simulink model "control_system"  (R2020b)
settings: Solver=FixedStepAuto  StartTime=0.0  StopTime=t_sim  FixedStep=Ts  RelTol=1e-2
values from neighbouring files (symbols this model uses):
  Hp = 10    [main_script.m]
  InitPosX = -2.4980e+03    (= -2498)    [main_script.m]
  InitPosY = -650.5503    [main_script.m]
  InitVelX = V0*cosd(InitYaw)    [main_script.m]
  InitVelY = V0*sind(InitYaw)    [main_script.m]
  InitYaw = 21    [main_script.m]
  lr = 1.592    [main_script.m]
  m = 1625    [main_script.m]
  Ts = 0.1    [main_script.m]
  V0 = 25    [main_script.m]
libraries: neural x856, simulink x1, autolibshared x1, drivingscenarioandsensors x1
(part 31 of 40)

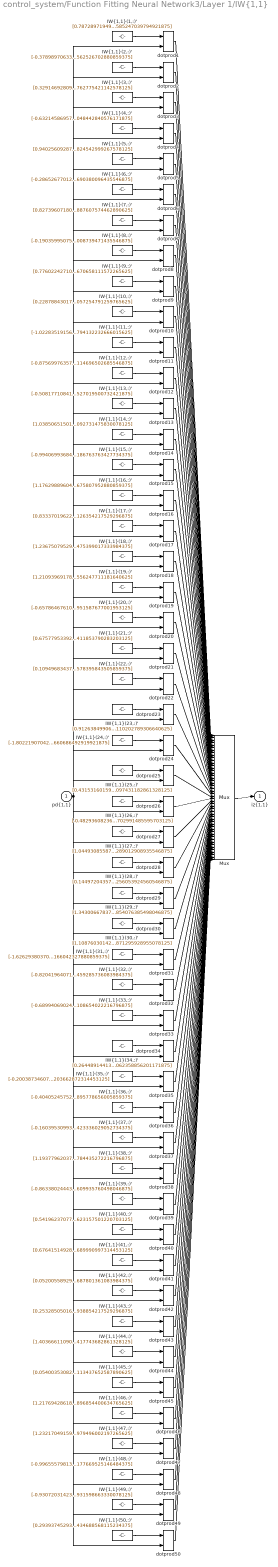
== system control_system/Function Fitting Neural Network3/Layer 1/IW{1,1} ==
  "pd{1,1}" : Inport  PortDimensions=9  SampleTime=0.1
      mask Display: e = 0.06;c1 = [120 230 180]/255;c2 = ([120 230 180]+0)/(256+128);c3 = ([120 230 180]+128)/(256+128);patch([0 1 1 0],[0 0 1 1],c1);patch([0 1 1 1-e 1-e 0+e],[0 0 1 1-e 0+e 0+e],c2);patch([0 0 1 1-e 0+e 0+e],[0 1 1 1-e 1-e 0+e],c3);plot([0 1 1 0 0],[0 0 1 1 0]);
  "IW{1,1}(1,:)'" : Constant  Value=[0.78728971949492476678500452180742286145687103271484375;0.352797731152850790881103648644057102501392364501953125;0.8265331890279414839284299887367524206638336181640625;-0.1863624056692552988234723443383700214326381683349609375;-0.7777782099348835576080318787717260420322418212890625;-0.5426301554164287832549007362104021012783050537109375;-0.6404421601342054071182019470143131911754608154296875;-0.99503704364510625612894045843859203159809112548828125;-0.948568198681023044827043122495524585247039794921875]
      mask Display: e = 0.06;c1 = [120 150 230]/255;c2 = ([120 150 230]+0)/383;c3 = ([120 150 230]+128)/383;patch([0 1 1 0],[0 0 1 1],c1);patch([0 1 1 1-e 1-e 0+e],[0 0 1 1-e 0+e 0+e],c2);patch([0 0 1 1-e 0+e 0+e],[0 1 1 1-e 1-e 0+e],c3);plot([0 1 1 0 0],[0 0 1 1 0]);disp('Weights');
  "IW{1,1}(10,:)'" : Constant  Value=[0.2287884301751469673380512404037290252745151519775390625;-0.0631161080977170330097436590222059749066829681396484375;1.0790651138932052521823834467795677483081817626953125;-0.738474613619092057348325397470034658908843994140625;0.0118735259410528148915631163617945276200771331787109375;1.1493716684892592017064316678442992269992828369140625;0.8580199635066418917261898968718014657497406005859375;0.1895198552495412636087479540947242639958858489990234375;-0.9068559161380724820133991670445539057254791259765625]
      mask Display: e = 0.06;c1 = [120 150 230]/255;c2 = ([120 150 230]+0)/383;c3 = ([120 150 230]+128)/383;patch([0 1 1 0],[0 0 1 1],c1);patch([0 1 1 1-e 1-e 0+e],[0 0 1 1-e 0+e 0+e],c2);patch([0 0 1 1-e 0+e 0+e],[0 1 1 1-e 1-e 0+e],c3);plot([0 1 1 0 0],[0 0 1 1 0]);disp('Weights');
  "IW{1,1}(11,:)'" : Constant  Value=[-1.0228351915632918345266944015747867524623870849609375;-0.021838659789676147238157710717132431454956531524658203125;-0.415484340574546917590481598381302319467067718505859375;-1.060341109567944695157848400413058698177337646484375;1.2054314419390748103211308261961676180362701416015625;-1.0443864348574185552109838681644760072231292724609375;-0.8779072415157027631238406684133224189281463623046875;0.349684007816375153065990843970212154090404510498046875;0.0266467695099608693765080857929206104017794132232666015625]
      mask Display: e = 0.06;c1 = [120 150 230]/255;c2 = ([120 150 230]+0)/383;c3 = ([120 150 230]+128)/383;patch([0 1 1 0],[0 0 1 1],c1);patch([0 1 1 1-e 1-e 0+e],[0 0 1 1-e 0+e 0+e],c2);patch([0 0 1 1-e 0+e 0+e],[0 1 1 1-e 1-e 0+e],c3);plot([0 1 1 0 0],[0 0 1 1 0]);disp('Weights');
  "IW{1,1}(12,:)'" : Constant  Value=[-0.875699763578115408790836227126419544219970703125;-0.242759821567909594985934518263093195855617523193359375;1.2159085613981057694132914548390544950962066650390625;0.4044163132053437692547959159128367900848388671875;1.07575999978741077001131998258642852306365966796875;1.8004386650346335674299780293949879705905914306640625;-0.9917103190571128212837948012747801840305328369140625;1.3494754673529085753358458532602526247501373291015625;-0.9851225876669171821475856631877832114696502685546875]
      mask Display: e = 0.06;c1 = [120 150 230]/255;c2 = ([120 150 230]+0)/383;c3 = ([120 150 230]+128)/383;patch([0 1 1 0],[0 0 1 1],c1);patch([0 1 1 1-e 1-e 0+e],[0 0 1 1-e 0+e 0+e],c2);patch([0 0 1 1-e 0+e 0+e],[0 1 1 1-e 1-e 0+e],c3);plot([0 1 1 0 0],[0 0 1 1 0]);disp('Weights');
  "IW{1,1}(13,:)'" : Constant  Value=[-0.50817710841719809788941120132221840322017669677734375;1.08852825196150693187746583134867250919342041015625;-1.3310195810328024901281196434865705668926239013671875;-1.041602136557479685308180705760605633258819580078125;-0.97705606452752336021916335084824822843074798583984375;-0.6948444334830787827428366654203273355960845947265625;-0.362171807844527238184895168160437606275081634521484375;0.1192369383747513833515796477513504214584827423095703125;0.290041715158442847677378040316398255527019500732421875]
      mask Display: e = 0.06;c1 = [120 150 230]/255;c2 = ([120 150 230]+0)/383;c3 = ([120 150 230]+128)/383;patch([0 1 1 0],[0 0 1 1],c1);patch([0 1 1 1-e 1-e 0+e],[0 0 1 1-e 0+e 0+e],c2);patch([0 0 1 1-e 0+e 0+e],[0 1 1 1-e 1-e 0+e],c3);plot([0 1 1 0 0],[0 0 1 1 0]);disp('Weights');
  "IW{1,1}(14,:)'" : Constant  Value=[1.0385065150165868619325237887096591293811798095703125;-0.0299341860920388953826165590044183772988617420196533203125;0.7451840663694848654330371573450975120067596435546875;-0.53186345138759227868519019466475583612918853759765625;-0.032742045322379752236852112901033251546323299407958984375;1.2450800939264377031889807767583988606929779052734375;1.1805822712498803550573711618199013173580169677734375;0.3130863479653560599302863920456729829311370849609375;0.2068094194929717410946778954894398339092731475830078125]
      mask Display: e = 0.06;c1 = [120 150 230]/255;c2 = ([120 150 230]+0)/383;c3 = ([120 150 230]+128)/383;patch([0 1 1 0],[0 0 1 1],c1);patch([0 1 1 1-e 1-e 0+e],[0 0 1 1-e 0+e 0+e],c2);patch([0 0 1 1-e 0+e 0+e],[0 1 1 1-e 1-e 0+e],c3);plot([0 1 1 0 0],[0 0 1 1 0]);disp('Weights');
  "IW{1,1}(15,:)'" : Constant  Value=[-0.99406993684322342286208140649250708520412445068359375;-0.334299503704392264591405137252877466380596160888671875;0.8578503214193753390048868823214434087276458740234375;-0.297048476488083579294396940895239822566509246826171875;-1.0704668818161728882643046745215542614459991455078125;-0.60807184451268858627059898935840465128421783447265625;-0.66391007727095929791261141872382722795009613037109375;1.66801104611655848231066556763835251331329345703125;-0.38683369041100712504288594573154114186763763427734375]
      mask Display: e = 0.06;c1 = [120 150 230]/255;c2 = ([120 150 230]+0)/383;c3 = ([120 150 230]+128)/383;patch([0 1 1 0],[0 0 1 1],c1);patch([0 1 1 1-e 1-e 0+e],[0 0 1 1-e 0+e 0+e],c2);patch([0 0 1 1-e 0+e 0+e],[0 1 1 1-e 1-e 0+e],c3);plot([0 1 1 0 0],[0 0 1 1 0]);disp('Weights');
  "IW{1,1}(16,:)'" : Constant  Value=[1.176298896048470599140500780777074396610260009765625;-0.8988232289150623888218660795246250927448272705078125;0.09615576773442553737414328907107119448482990264892578125;0.48788471027654944922602453516446985304355621337890625;1.037047709591436994713831154513172805309295654296875;0.55055285364358841349030626588501036167144775390625;-0.17909145298814654889696384998387657105922698974609375;0.81145522342693199302487983004539273679256439208984375;0.021295651159626081960762888911631307564675807952880859375]
      mask Display: e = 0.06;c1 = [120 150 230]/255;c2 = ([120 150 230]+0)/383;c3 = ([120 150 230]+128)/383;patch([0 1 1 0],[0 0 1 1],c1);patch([0 1 1 1-e 1-e 0+e],[0 0 1 1-e 0+e 0+e],c2);patch([0 0 1 1-e 0+e 0+e],[0 1 1 1-e 1-e 0+e],c3);plot([0 1 1 0 0],[0 0 1 1 0]);disp('Weights');
  "IW{1,1}(17,:)'" : Constant  Value=[0.83337019622696739684641897838446311652660369873046875;-0.36366566717185555557279030836070887744426727294921875;-0.96023270638495639150988836263422854244709014892578125;1.2783373677316156591388107699458487331867218017578125;0.8916276331235633012539665287476964294910430908203125;-0.6694170731239468263851222218363545835018157958984375;-0.925192516466152081733298473409377038478851318359375;-1.052006199283979537284494654159061610698699951171875;-0.7764706210752112536255253871786408126354217529296875]
      mask Display: e = 0.06;c1 = [120 150 230]/255;c2 = ([120 150 230]+0)/383;c3 = ([120 150 230]+128)/383;patch([0 1 1 0],[0 0 1 1],c1);patch([0 1 1 1-e 1-e 0+e],[0 0 1 1-e 0+e 0+e],c2);patch([0 0 1 1-e 0+e 0+e],[0 1 1 1-e 1-e 0+e],c3);plot([0 1 1 0 0],[0 0 1 1 0]);disp('Weights');
  "IW{1,1}(18,:)'" : Constant  Value=[1.236750795296624350072534070932306349277496337890625;-0.55986879173246772989358532868209294974803924560546875;-1.3800915711518084716402654521516524255275726318359375;1.3289904008938917545634694761247374117374420166015625;0.60327067881495100021282951274770312011241912841796875;-0.4150673095081656160942884525866247713565826416015625;-0.019363883654753132057546594069208367727696895599365234375;0.1294585767502997308842083157287561334669589996337890625;-0.74106167458830130012614745282917283475399017333984375]
      mask Display: e = 0.06;c1 = [120 150 230]/255;c2 = ([120 150 230]+0)/383;c3 = ([120 150 230]+128)/383;patch([0 1 1 0],[0 0 1 1],c1);patch([0 1 1 1-e 1-e 0+e],[0 0 1 1-e 0+e 0+e],c2);patch([0 0 1 1-e 0+e 0+e],[0 1 1 1-e 1-e 0+e],c3);plot([0 1 1 0 0],[0 0 1 1 0]);disp('Weights');
  "IW{1,1}(19,:)'" : Constant  Value=[1.2109396917827270900858138702460564672946929931640625;0.1326857718800483476595530873964889906346797943115234375;-0.465325794397773273569640650748624466359615325927734375;-0.53881885042031452126565227445098571479320526123046875;-0.8667873778604668899561147554777562618255615234375;-0.1324460904740631661535843477395246736705303192138671875;-0.6026871578635122350675601410330273211002349853515625;0.2041421396899969764593407717256923206150531768798828125;1.1937448304855708958172044731327332556247711181640625]
      mask Display: e = 0.06;c1 = [120 150 230]/255;c2 = ([120 150 230]+0)/383;c3 = ([120 150 230]+128)/383;patch([0 1 1 0],[0 0 1 1],c1);patch([0 1 1 1-e 1-e 0+e],[0 0 1 1-e 0+e 0+e],c2);patch([0 0 1 1-e 0+e 0+e],[0 1 1 1-e 1-e 0+e],c3);plot([0 1 1 0 0],[0 0 1 1 0]);disp('Weights');
  "IW{1,1}(2,:)'" : Constant  Value=[-0.378989706335502607448262324396637268364429473876953125;-1.1437056077678295906707717222161591053009033203125;0.330358132573418228350448089258861728012561798095703125;-0.476080786756290341710240454631275497376918792724609375;-0.4363164287721887912852025692700408399105072021484375;-0.63772136886470409677940551773644983768463134765625;-1.174846406412093369198146319831721484661102294921875;-0.77474853404004928592030410072766244411468505859375;-0.2296675389268350853111400056150159798562526702880859375]
      mask Display: e = 0.06;c1 = [120 150 230]/255;c2 = ([120 150 230]+0)/383;c3 = ([120 150 230]+128)/383;patch([0 1 1 0],[0 0 1 1],c1);patch([0 1 1 1-e 1-e 0+e],[0 0 1 1-e 0+e 0+e],c2);patch([0 0 1 1-e 0+e 0+e],[0 1 1 1-e 1-e 0+e],c3);plot([0 1 1 0 0],[0 0 1 1 0]);disp('Weights');
  "IW{1,1}(20,:)'" : Constant  Value=[-0.65786467610956089746565567111247219145298004150390625;1.362933438760308479942295889486558735370635986328125;0.210346089395960611501124049027566798031330108642578125;-0.7030459458053137655753062063013203442096710205078125;0.63733479975609863554808498520287685096263885498046875;-0.7983018398063055354185735268401913344860076904296875;0.648857536128780498785317831789143383502960205078125;0.8394757099670868694119008068810217082500457763671875;-0.52279242792795888039592000495758838951587677001953125]
      mask Display: e = 0.06;c1 = [120 150 230]/255;c2 = ([120 150 230]+0)/383;c3 = ([120 150 230]+128)/383;patch([0 1 1 0],[0 0 1 1],c1);patch([0 1 1 1-e 1-e 0+e],[0 0 1 1-e 0+e 0+e],c2);patch([0 0 1 1-e 0+e 0+e],[0 1 1 1-e 1-e 0+e],c3);plot([0 1 1 0 0],[0 0 1 1 0]);disp('Weights');
  "IW{1,1}(21,:)'" : Constant  Value=[0.67577953392096989926329797526705078780651092529296875;0.8608869950072242094307739534997381269931793212890625;-0.11469898640935526079598361093303537927567958831787109375;1.1193380407867741244132275824085809290409088134765625;-0.9683403733384603473410834340029396116733551025390625;0.027391112412877567650060228743313928134739398956298828125;-1.209926726376689298803057681652717292308807373046875;-0.268730649947182820280744408591999672353267669677734375;-0.8212758063260576779640587119502015411853790283203125]
      mask Display: e = 0.06;c1 = [120 150 230]/255;c2 = ([120 150 230]+0)/383;c3 = ([120 150 230]+128)/383;patch([0 1 1 0],[0 0 1 1],c1);patch([0 1 1 1-e 1-e 0+e],[0 0 1 1-e 0+e 0+e],c2);patch([0 0 1 1-e 0+e 0+e],[0 1 1 1-e 1-e 0+e],c3);plot([0 1 1 0 0],[0 0 1 1 0]);disp('Weights');
  "IW{1,1}(22,:)'" : Constant  Value=[0.10949683437770142691025654357872554101049900054931640625;0.87280978510004214587780779766035266220569610595703125;-1.0316109104847950295180680768680758774280548095703125;0.9729898005523214266077047795988619327545166015625;1.0304574213938497706521957297809422016143798828125;-0.341709897445362897894227671713451854884624481201171875;-0.6454097992064846689430623882799409329891204833984375;-0.656223486076811468592495657503604888916015625;0.2604852028852560064109411541721783578395843505859375]
      mask Display: e = 0.06;c1 = [120 150 230]/255;c2 = ([120 150 230]+0)/383;c3 = ([120 150 230]+128)/383;patch([0 1 1 0],[0 0 1 1],c1);patch([0 1 1 1-e 1-e 0+e],[0 0 1 1-e 0+e 0+e],c2);patch([0 0 1 1-e 0+e 0+e],[0 1 1 1-e 1-e 0+e],c3);plot([0 1 1 0 0],[0 0 1 1 0]);disp('Weights');
  "IW{1,1}(23,:)'" : Constant  Value=[0.912638499065945740795768870157189667224884033203125;0.62788843775751457254585830014548264443874359130859375;-0.11544045247414332078239596057755989022552967071533203125;0.72876930448921173333332035326748155057430267333984375;0.0930837705597644948785074348052148707211017608642578125;0.70534305814777942256199594339705072343349456787109375;0.79724782708528263430736160444212146103382110595703125;1.5542498026142135270077915265574119985103607177734375;-0.0814864679916317558028282519444474019110202789306640625]
      mask Display: e = 0.06;c1 = [120 150 230]/255;c2 = ([120 150 230]+0)/383;c3 = ([120 150 230]+128)/383;patch([0 1 1 0],[0 0 1 1],c1);patch([0 1 1 1-e 1-e 0+e],[0 0 1 1-e 0+e 0+e],c2);patch([0 0 1 1-e 0+e 0+e],[0 1 1 1-e 1-e 0+e],c3);plot([0 1 1 0 0],[0 0 1 1 0]);disp('Weights');
  "IW{1,1}(24,:)'" : Constant  Value=[-1.802219070424301516908371922909282147884368896484375;-0.340985615024179289367367573504452593624591827392578125;-0.5377858984214862747563756784074939787387847900390625;-1.515689046597109790326385336811654269695281982421875;0.51434483958638843592581224584137089550495147705078125;-0.1567876230668934223189125987119041383266448974609375;0.351340893838307299912315784240490756928920745849609375;1.368712963354658196379887158400379121303558349609375;-0.66279873807852573985854860438848845660686492919921875]
      mask Display: e = 0.06;c1 = [120 150 230]/255;c2 = ([120 150 230]+0)/383;c3 = ([120 150 230]+128)/383;patch([0 1 1 0],[0 0 1 1],c1);patch([0 1 1 1-e 1-e 0+e],[0 0 1 1-e 0+e 0+e],c2);patch([0 0 1 1-e 0+e 0+e],[0 1 1 1-e 1-e 0+e],c3);plot([0 1 1 0 0],[0 0 1 1 0]);disp('Weights');
  "IW{1,1}(25,:)'" : Constant  Value=[0.43153160159828851671903748865588568150997161865234375;-0.77360038084864990448608068618341349065303802490234375;-1.18295318629940737764627556316554546356201171875;-0.433606385185640819113217503399937413632869720458984375;-0.2244183057689046467686466712621040642261505126953125;-0.7321900135293717415407854787190444767475128173828125;-0.451425117568696077086087825591675937175750732421875;1.1856571858869806579406258606468327343463897705078125;0.04425940707458864142864740642835386097431182861328125]
      mask Display: e = 0.06;c1 = [120 150 230]/255;c2 = ([120 150 230]+0)/383;c3 = ([120 150 230]+128)/383;patch([0 1 1 0],[0 0 1 1],c1);patch([0 1 1 1-e 1-e 0+e],[0 0 1 1-e 0+e 0+e],c2);patch([0 0 1 1-e 0+e 0+e],[0 1 1 1-e 1-e 0+e],c3);plot([0 1 1 0 0],[0 0 1 1 0]);disp('Weights');
  "IW{1,1}(26,:)'" : Constant  Value=[-0.482936082364363639118920445980620570480823516845703125;-0.9309568746589584886663715224131010472774505615234375;-0.1503448104672455432062605495957541279494762420654296875;-1.198029994378850826564075759961269795894622802734375;0.259575336572962889203353142875130288302898406982421875;0.27904855673582318331682472489774227142333984375;-0.50645491575020995522748989969841204583644866943359375;0.62272600542499245701577592626563273370265960693359375;-1.202204106531607141761242019128985702991485595703125]
      mask Display: e = 0.06;c1 = [120 150 230]/255;c2 = ([120 150 230]+0)/383;c3 = ([120 150 230]+128)/383;patch([0 1 1 0],[0 0 1 1],c1);patch([0 1 1 1-e 1-e 0+e],[0 0 1 1-e 0+e 0+e],c2);patch([0 0 1 1-e 0+e 0+e],[0 1 1 1-e 1-e 0+e],c3);plot([0 1 1 0 0],[0 0 1 1 0]);disp('Weights');
  "IW{1,1}(27,:)'" : Constant  Value=[1.044930855879160791488402537652291357517242431640625;-0.860944056842925409256395141710527241230010986328125;0.887825241736790449209593134582974016666412353515625;0.427993292709983375043947262383881025016307830810546875;-0.457723346034051792319274909459636546671390533447265625;-0.55042069308471652799852336102048866450786590576171875;-0.87332778872113137058619258823455311357975006103515625;-0.6366049352812364059417404860141687095165252685546875;0.70842194831802440813106613859417848289012908935546875]
      mask Display: e = 0.06;c1 = [120 150 230]/255;c2 = ([120 150 230]+0)/383;c3 = ([120 150 230]+128)/383;patch([0 1 1 0],[0 0 1 1],c1);patch([0 1 1 1-e 1-e 0+e],[0 0 1 1-e 0+e 0+e],c2);patch([0 0 1 1-e 0+e 0+e],[0 1 1 1-e 1-e 0+e],c3);plot([0 1 1 0 0],[0 0 1 1 0]);disp('Weights');
  "IW{1,1}(28,:)'" : Constant  Value=[0.144972043576537090725508960531442426145076751708984375;0.1541953436889172690538174492758116684854030609130859375;-0.77822769384765655420466146097169257700443267822265625;-1.0198035630015633845601996654295362532138824462890625;-0.51659780456091886069458496422157622873783111572265625;1.39939210966581573103439950500614941120147705078125;0.295882266856562381462936173193156719207763671875;1.0654792493903155747858590984833426773548126220703125;0.641300014924847783248651467147283256053924560546875]
      mask Display: e = 0.06;c1 = [120 150 230]/255;c2 = ([120 150 230]+0)/383;c3 = ([120 150 230]+128)/383;patch([0 1 1 0],[0 0 1 1],c1);patch([0 1 1 1-e 1-e 0+e],[0 0 1 1-e 0+e 0+e],c2);patch([0 0 1 1-e 0+e 0+e],[0 1 1 1-e 1-e 0+e],c3);plot([0 1 1 0 0],[0 0 1 1 0]);disp('Weights');
  "IW{1,1}(29,:)'" : Constant  Value=[1.3430066783716971823281483011669479310512542724609375;-0.8969042973177840938348026611492969095706939697265625;-1.076092110823586356360692661837674677371978759765625;0.244234872350051868128417709158384241163730621337890625;0.495632237070989634108997279327013529837131500244140625;-0.31289164058760310371809509888407774269580841064453125;-0.912975658702446679626518744044005870819091796875;0.0809968678519148443939457138185389339923858642578125;0.397991863783186516911882790736854076385498046875]
      mask Display: e = 0.06;c1 = [120 150 230]/255;c2 = ([120 150 230]+0)/383;c3 = ([120 150 230]+128)/383;patch([0 1 1 0],[0 0 1 1],c1);patch([0 1 1 1-e 1-e 0+e],[0 0 1 1-e 0+e 0+e],c2);patch([0 0 1 1-e 0+e 0+e],[0 1 1 1-e 1-e 0+e],c3);plot([0 1 1 0 0],[0 0 1 1 0]);disp('Weights');
  "IW{1,1}(3,:)'" : Constant  Value=[0.3291469280906638150696608136058785021305084228515625;0.62737660797549354985136460527428425848484039306640625;0.78915346814299869304676349202054552733898162841796875;-0.90552136457697385285570135238231159746646881103515625;0.257465585146909037295159805580624379217624664306640625;0.221382776389055069277134180083521641790866851806640625;1.4252850062237729655834073128062300384044647216796875;-0.69989724392903751581940241521806456148624420166015625;0.20729749308358613735236986030940897762775421142578125]
      mask Display: e = 0.06;c1 = [120 150 230]/255;c2 = ([120 150 230]+0)/383;c3 = ([120 150 230]+128)/383;patch([0 1 1 0],[0 0 1 1],c1);patch([0 1 1 1-e 1-e 0+e],[0 0 1 1-e 0+e 0+e],c2);patch([0 0 1 1-e 0+e 0+e],[0 1 1 1-e 1-e 0+e],c3);plot([0 1 1 0 0],[0 0 1 1 0]);disp('Weights');
  "IW{1,1}(30,:)'" : Constant  Value=[1.108760301421545246824962305254302918910980224609375;0.86207759324852251126003466197289526462554931640625;-0.11670050893409382453125289202944259159266948699951171875;1.2386076034523905153861278449767269194126129150390625;-1.0526726240503554432592636658228002488613128662109375;1.1240606375888670953600012580864131450653076171875;0.92538279206566487200547044267295859754085540771484375;-1.3685636484095333731403343335841782391071319580078125;-0.69779752491048718798793970563565380871295928955078125]
      mask Display: e = 0.06;c1 = [120 150 230]/255;c2 = ([120 150 230]+0)/383;c3 = ([120 150 230]+128)/383;patch([0 1 1 0],[0 0 1 1],c1);patch([0 1 1 1-e 1-e 0+e],[0 0 1 1-e 0+e 0+e],c2);patch([0 0 1 1-e 0+e 0+e],[0 1 1 1-e 1-e 0+e],c3);plot([0 1 1 0 0],[0 0 1 1 0]);disp('Weights');
  "IW{1,1}(31,:)'" : Constant  Value=[-1.6262938037064917917717821183032356202602386474609375;-0.347778459901182335212155294357216916978359222412109375;0.83231871936962031899298608550452627241611480712890625;-1.122571461750564214554515274357981979846954345703125;1.039097624203837444412101831403560936450958251953125;-0.81297977449732883314936771057546138763427734375;1.113158335871994975008192341192625463008880615234375;-0.1408702915339343775258384994231164455413818359375;-0.031547675269102126716092016067705117166042327880859375]
      mask Display: e = 0.06;c1 = [120 150 230]/255;c2 = ([120 150 230]+0)/383;c3 = ([120 150 230]+128)/383;patch([0 1 1 0],[0 0 1 1],c1);patch([0 1 1 1-e 1-e 0+e],[0 0 1 1-e 0+e 0+e],c2);patch([0 0 1 1-e 0+e 0+e],[0 1 1 1-e 1-e 0+e],c3);plot([0 1 1 0 0],[0 0 1 1 0]);disp('Weights');
  "IW{1,1}(32,:)'" : Constant  Value=[-0.82041964071189787954807570713455788791179656982421875;-0.32324692831648238477981749383616261184215545654296875;0.6458209200762670132434095648932270705699920654296875;0.23384694042951437165100969650666229426860809326171875;-1.291500322629459684975472555379383265972137451171875;-1.5974304191525749985203219694085419178009033203125;0.444373258878406340866007440126850269734859466552734375;1.57149179936640681631843108334578573703765869140625;0.269491929332904278648896934100775979459285736083984375]
      mask Display: e = 0.06;c1 = [120 150 230]/255;c2 = ([120 150 230]+0)/383;c3 = ([120 150 230]+128)/383;patch([0 1 1 0],[0 0 1 1],c1);patch([0 1 1 1-e 1-e 0+e],[0 0 1 1-e 0+e 0+e],c2);patch([0 0 1 1-e 0+e 0+e],[0 1 1 1-e 1-e 0+e],c3);plot([0 1 1 0 0],[0 0 1 1 0]);disp('Weights');
  "IW{1,1}(33,:)'" : Constant  Value=[-0.689940690243980636608966960920952260494232177734375;-1.4101558786294583480724895707680843770503997802734375;0.1630877244993971242337238436448387801647186279296875;-1.7669812635201058714784494441119022667407989501953125;-0.482624421254764346400634167366661131381988525390625;-0.9612055055403947445569201590842567384243011474609375;1.3015624416982609634629852735088206827640533447265625;0.0875738032916208719580453134767594747245311737060546875;0.040220794334714475570802250103952246718108654022216796875]
      mask Display: e = 0.06;c1 = [120 150 230]/255;c2 = ([120 150 230]+0)/383;c3 = ([120 150 230]+128)/383;patch([0 1 1 0],[0 0 1 1],c1);patch([0 1 1 1-e 1-e 0+e],[0 0 1 1-e 0+e 0+e],c2);patch([0 0 1 1-e 0+e 0+e],[0 1 1 1-e 1-e 0+e],c3);plot([0 1 1 0 0],[0 0 1 1 0]);disp('Weights');
  "IW{1,1}(34,:)'" : Constant  Value=[0.264489144130551523392824719849159009754657745361328125;-0.11668913145246741225324882407221593894064426422119140625;0.60220127682401358715225114792701788246631622314453125;1.7380237708569612475884014202165417373180389404296875;0.6104130038792170420691718391026370227336883544921875;-1.70710467850310987358852798934094607830047607421875;-0.92955480038042848089929748311988078057765960693359375;1.5937912860225769140498641718295402824878692626953125;1.4518733032150279438354800731758587062358856201171875]
      mask Display: e = 0.06;c1 = [120 150 230]/255;c2 = ([120 150 230]+0)/383;c3 = ([120 150 230]+128)/383;patch([0 1 1 0],[0 0 1 1],c1);patch([0 1 1 1-e 1-e 0+e],[0 0 1 1-e 0+e 0+e],c2);patch([0 0 1 1-e 0+e 0+e],[0 1 1 1-e 1-e 0+e],c3);plot([0 1 1 0 0],[0 0 1 1 0]);disp('Weights');
  "IW{1,1}(35,:)'" : Constant  Value=[-0.200387346072296856913652618459309451282024383544921875;0.478387526639784843585090357009903527796268463134765625;1.19705813553185880238061145064420998096466064453125;-1.525560920857229607605631827027536928653717041015625;-1.11857885098643095034276484511792659759521484375;2.28596493044082382795068042469210922718048095703125;-0.32697021581169305459724228057893924415111541748046875;0.1161743373023399750199047275600605644285678863525390625;0.9455134287433129003375142929144203662872314453125]
      mask Display: e = 0.06;c1 = [120 150 230]/255;c2 = ([120 150 230]+0)/383;c3 = ([120 150 230]+128)/383;patch([0 1 1 0],[0 0 1 1],c1);patch([0 1 1 1-e 1-e 0+e],[0 0 1 1-e 0+e 0+e],c2);patch([0 0 1 1-e 0+e 0+e],[0 1 1 1-e 1-e 0+e],c3);plot([0 1 1 0 0],[0 0 1 1 0]);disp('Weights');
  "IW{1,1}(36,:)'" : Constant  Value=[-0.4040524575299941911765699842362664639949798583984375;0.56950173003886794820260774940834380686283111572265625;-0.309069682024796510422248729810235090553760528564453125;1.174907768493887783023410520399920642375946044921875;-0.76016435248717650896566055962466634809970855712890625;0.463070298319331830061429400302586145699024200439453125;-0.71977379111322481453072441581753082573413848876953125;0.1662797156150146171693648966538603417575359344482421875;1.231310054411932863871470544836483895778656005859375]
      mask Display: e = 0.06;c1 = [120 150 230]/255;c2 = ([120 150 230]+0)/383;c3 = ([120 150 230]+128)/383;patch([0 1 1 0],[0 0 1 1],c1);patch([0 1 1 1-e 1-e 0+e],[0 0 1 1-e 0+e 0+e],c2);patch([0 0 1 1-e 0+e 0+e],[0 1 1 1-e 1-e 0+e],c3);plot([0 1 1 0 0],[0 0 1 1 0]);disp('Weights');
  "IW{1,1}(37,:)'" : Constant  Value=[-0.160395309938668961802221701873349957168102264404296875;0.410351798316771709806971557554788887500762939453125;1.0788402606665403737906672176904976367950439453125;-0.32839166335755642922578090292518027126789093017578125;-1.0325028530439583906996858786442317068576812744140625;-0.33651519126705686790756999471341259777545928955078125;0.00718425054981363005179861858096046489663422107696533203125;-0.87535165476770548931284565696842037141323089599609375;0.93976986860059719131044175810529850423336029052734375]
      mask Display: e = 0.06;c1 = [120 150 230]/255;c2 = ([120 150 230]+0)/383;c3 = ([120 150 230]+128)/383;patch([0 1 1 0],[0 0 1 1],c1);patch([0 1 1 1-e 1-e 0+e],[0 0 1 1-e 0+e 0+e],c2);patch([0 0 1 1-e 0+e 0+e],[0 1 1 1-e 1-e 0+e],c3);plot([0 1 1 0 0],[0 0 1 1 0]);disp('Weights');
  "IW{1,1}(38,:)'" : Constant  Value=[1.1937796203738368916447143419645726680755615234375;1.230789293167344755630665531498380005359649658203125;0.07832258154244080283756801463823649100959300994873046875;1.5392943653869954889756854754523374140262603759765625;1.5136918318591983112497700858511961996555328369140625;-0.241736218705538796758247599427704699337482452392578125;0.2867327195668918360382804166874848306179046630859375;-1.2139662037220404489090697097708471119403839111328125;0.79571289507152431763614686133223585784435272216796875]
      mask Display: e = 0.06;c1 = [120 150 230]/255;c2 = ([120 150 230]+0)/383;c3 = ([120 150 230]+128)/383;patch([0 1 1 0],[0 0 1 1],c1);patch([0 1 1 1-e 1-e 0+e],[0 0 1 1-e 0+e 0+e],c2);patch([0 0 1 1-e 0+e 0+e],[0 1 1 1-e 1-e 0+e],c3);plot([0 1 1 0 0],[0 0 1 1 0]);disp('Weights');
  "IW{1,1}(39,:)'" : Constant  Value=[-0.86338024443859662238054397676023654639720916748046875;0.86905909058558783453207752245361916720867156982421875;0.578888775818624079505525514832697808742523193359375;-1.474862708423287482872865439276210963726043701171875;1.095471724648996225681685245945118367671966552734375;-0.70623810094509276158447619309299625456333160400390625;-1.1869666187459351203159485521609894931316375732421875;0.206434423646733034019007391179911792278289794921875;-0.91825459226975592041952722865971736609935760498046875]
      mask Display: e = 0.06;c1 = [120 150 230]/255;c2 = ([120 150 230]+0)/383;c3 = ([120 150 230]+128)/383;patch([0 1 1 0],[0 0 1 1],c1);patch([0 1 1 1-e 1-e 0+e],[0 0 1 1-e 0+e 0+e],c2);patch([0 0 1 1-e 0+e 0+e],[0 1 1 1-e 1-e 0+e],c3);plot([0 1 1 0 0],[0 0 1 1 0]);disp('Weights');
  "IW{1,1}(4,:)'" : Constant  Value=[-0.6321458695752950607271714034141041338443756103515625;0.54688250895527812378560383876902051270008087158203125;0.1788397574811165513519739533876418136060237884521484375;0.59342891536845499000918380261282436549663543701171875;0.76115013925244967563088493989198468625545501708984375;1.3158823761126641205265741518815048038959503173828125;1.2724410126391259012734735733829438686370849609375;1.7966390556129059330459085686015896499156951904296875;-0.0220531766669407151837400959948354284279048442840576171875]
      mask Display: e = 0.06;c1 = [120 150 230]/255;c2 = ([120 150 230]+0)/383;c3 = ([120 150 230]+128)/383;patch([0 1 1 0],[0 0 1 1],c1);patch([0 1 1 1-e 1-e 0+e],[0 0 1 1-e 0+e 0+e],c2);patch([0 0 1 1-e 0+e 0+e],[0 1 1 1-e 1-e 0+e],c3);plot([0 1 1 0 0],[0 0 1 1 0]);disp('Weights');
  "IW{1,1}(40,:)'" : Constant  Value=[0.5419623707778138399504541666829027235507965087890625;0.1950556215816010297015026253575342707335948944091796875;1.078199970146870523279858389287255704402923583984375;-1.674137574591714194838232288020662963390350341796875;-0.7880522431413308215297774950158782303333282470703125;0.68010644380544338361005429760552942752838134765625;0.4078215424324758142660130033618770539760589599609375;-2.306607321515167452474770470871590077877044677734375;-0.12174585245644194142489169507825863547623157501220703125]
      mask Display: e = 0.06;c1 = [120 150 230]/255;c2 = ([120 150 230]+0)/383;c3 = ([120 150 230]+128)/383;patch([0 1 1 0],[0 0 1 1],c1);patch([0 1 1 1-e 1-e 0+e],[0 0 1 1-e 0+e 0+e],c2);patch([0 0 1 1-e 0+e 0+e],[0 1 1 1-e 1-e 0+e],c3);plot([0 1 1 0 0],[0 0 1 1 0]);disp('Weights');
  "IW{1,1}(41,:)'" : Constant  Value=[0.67641514928419399499404107700684107840061187744140625;-0.8238474701929126009503079330897890031337738037109375;0.7852656164367346480759124460746534168720245361328125;-1.104985223708661923325280440622009336948394775390625;0.8669948164997738349057954110321588814258575439453125;-0.1704696961773134178397270943605690263211727142333984375;0.568046795494847600593857350759208202362060546875;-0.34251139207962777444294033557525835931301116943359375;-0.5210710874334314457456684976932592689990997314453125]
      mask Display: e = 0.06;c1 = [120 150 230]/255;c2 = ([120 150 230]+0)/383;c3 = ([120 150 230]+128)/383;patch([0 1 1 0],[0 0 1 1],c1);patch([0 1 1 1-e 1-e 0+e],[0 0 1 1-e 0+e 0+e],c2);patch([0 0 1 1-e 0+e 0+e],[0 1 1 1-e 1-e 0+e],c3);plot([0 1 1 0 0],[0 0 1 1 0]);disp('Weights');
  "IW{1,1}(42,:)'" : Constant  Value=[0.052005589294320149484907034320713137276470661163330078125;-0.90943826081045686660075944018899463117122650146484375;0.693083964699585219904065525042824447154998779296875;-0.0306181895012466454009114613654674030840396881103515625;-1.029794535030280844267736028996296226978302001953125;1.4265242294115925147934831329621374607086181640625;-1.2134293112742839948481332612573169171810150146484375;-0.14285369445769280360991615452803671360015869140625;-0.2337878360452552983783647277959971688687801361083984375]
      mask Display: e = 0.06;c1 = [120 150 230]/255;c2 = ([120 150 230]+0)/383;c3 = ([120 150 230]+128)/383;patch([0 1 1 0],[0 0 1 1],c1);patch([0 1 1 1-e 1-e 0+e],[0 0 1 1-e 0+e 0+e],c2);patch([0 0 1 1-e 0+e 0+e],[0 1 1 1-e 1-e 0+e],c3);plot([0 1 1 0 0],[0 0 1 1 0]);disp('Weights');
  "IW{1,1}(43,:)'" : Constant  Value=[0.253285050161697722348463912567240186035633087158203125;0.80455178080571954080113528107176534831523895263671875;0.00586296148288324714403785264948965050280094146728515625;0.416382999142569099060295911840512417256832122802734375;-1.3325808266979117799877485595061443746089935302734375;-0.199357366934553692505716071536880917847156524658203125;-0.98699903008132217063774760390515439212322235107421875;0.86596978278439629139739963648025877773761749267578125;-0.592039337966045575711859783041290938854217529296875]
      mask Display: e = 0.06;c1 = [120 150 230]/255;c2 = ([120 150 230]+0)/383;c3 = ([120 150 230]+128)/383;patch([0 1 1 0],[0 0 1 1],c1);patch([0 1 1 1-e 1-e 0+e],[0 0 1 1-e 0+e 0+e],c2);patch([0 0 1 1-e 0+e 0+e],[0 1 1 1-e 1-e 0+e],c3);plot([0 1 1 0 0],[0 0 1 1 0]);disp('Weights');
  "IW{1,1}(44,:)'" : Constant  Value=[1.4036661109019077375847928124130703508853912353515625;0.46243411607628714943274417237262241542339324951171875;-0.388355948716691268263190295328968204557895660400390625;0.08519612019570575733862227707504644058644771575927734375;0.5508784185981874248483336486970074474811553955078125;0.6600291717375321720595593433245085179805755615234375;-0.7760012903809980766567377941100858151912689208984375;-0.29527434493454174369020392987295053899288177490234375;0.1619492533726245853120673245939542539417743682861328125]
      mask Display: e = 0.06;c1 = [120 150 230]/255;c2 = ([120 150 230]+0)/383;c3 = ([120 150 230]+128)/383;patch([0 1 1 0],[0 0 1 1],c1);patch([0 1 1 1-e 1-e 0+e],[0 0 1 1-e 0+e 0+e],c2);patch([0 0 1 1-e 0+e 0+e],[0 1 1 1-e 1-e 0+e],c3);plot([0 1 1 0 0],[0 0 1 1 0]);disp('Weights');
  "IW{1,1}(45,:)'" : Constant  Value=[0.054003530822353019991144407185856834985315799713134765625;-0.7190132178875867641210106739890761673450469970703125;0.37819488489305097544956879573874175548553466796875;0.75355546016111729645814421019167639315128326416015625;0.44370790430326134679006599981221370398998260498046875;-0.709936431995932704097640453255735337734222412109375;-1.1461919921726171356368695342098362743854522705078125;0.800595455626574192820044117979705333709716796875;0.99754143380247572991947890841402113437652587890625]
      mask Display: e = 0.06;c1 = [120 150 230]/255;c2 = ([120 150 230]+0)/383;c3 = ([120 150 230]+128)/383;patch([0 1 1 0],[0 0 1 1],c1);patch([0 1 1 1-e 1-e 0+e],[0 0 1 1-e 0+e 0+e],c2);patch([0 0 1 1-e 0+e 0+e],[0 1 1 1-e 1-e 0+e],c3);plot([0 1 1 0 0],[0 0 1 1 0]);disp('Weights');
  "IW{1,1}(46,:)'" : Constant  Value=[1.2176942861808093265807428906555287539958953857421875;-0.2306704003439855321655471698250039480626583099365234375;-0.837885093416974147118025939562357962131500244140625;1.3581183357975390446625851836870424449443817138671875;0.0171206448053236835737944687707567936740815639495849609375;-0.44368483558002547173515495160245336592197418212890625;-1.011310446342665869678967283107340335845947265625;0.4686118622362638319600591785274446010589599609375;0.1100616896796785815215713455472723580896854400634765625]
      mask Display: e = 0.06;c1 = [120 150 230]/255;c2 = ([120 150 230]+0)/383;c3 = ([120 150 230]+128)/383;patch([0 1 1 0],[0 0 1 1],c1);patch([0 1 1 1-e 1-e 0+e],[0 0 1 1-e 0+e 0+e],c2);patch([0 0 1 1-e 0+e 0+e],[0 1 1 1-e 1-e 0+e],c3);plot([0 1 1 0 0],[0 0 1 1 0]);disp('Weights');
  "IW{1,1}(47,:)'" : Constant  Value=[1.232170491594959838010936437058262526988983154296875;-0.637608585363382385224895188002847135066986083984375;0.82397041188962649727045572944916784763336181640625;-1.0623012055518186169678074293187819421291351318359375;0.85759259558929823441530970740132033824920654296875;-0.158615357228967412961395666570751927793025970458984375;0.10049397403217685820209226221777498722076416015625;0.37062571004901112559082321240566670894622802734375;-0.137417487475233690563669597395346499979496002197265625]
      mask Display: e = 0.06;c1 = [120 150 230]/255;c2 = ([120 150 230]+0)/383;c3 = ([120 150 230]+128)/383;patch([0 1 1 0],[0 0 1 1],c1);patch([0 1 1 1-e 1-e 0+e],[0 0 1 1-e 0+e 0+e],c2);patch([0 0 1 1-e 0+e 0+e],[0 1 1 1-e 1-e 0+e],c3);plot([0 1 1 0 0],[0 0 1 1 0]);disp('Weights');
  "IW{1,1}(48,:)'" : Constant  Value=[-0.99655579813050376714045341941528022289276123046875;0.65771268442165686796130330549203790724277496337890625;0.85451265623490268996675922608119435608386993408203125;0.866575583683616645913616594043560326099395751953125;0.341105018364091183702413445644197054207324981689453125;0.504243458671222555267377174459397792816162109375;-1.1449037906206485093463243174483068287372589111328125;0.2206360035472175462611943430601968429982662200927734375;0.1902191501945905416359750006449758075177669525146484375]
      mask Display: e = 0.06;c1 = [120 150 230]/255;c2 = ([120 150 230]+0)/383;c3 = ([120 150 230]+128)/383;patch([0 1 1 0],[0 0 1 1],c1);patch([0 1 1 1-e 1-e 0+e],[0 0 1 1-e 0+e 0+e],c2);patch([0 0 1 1-e 0+e 0+e],[0 1 1 1-e 1-e 0+e],c3);plot([0 1 1 0 0],[0 0 1 1 0]);disp('Weights');
  "IW{1,1}(49,:)'" : Constant  Value=[-0.93072031423096224234114970386144705116748809814453125;0.314452546869901039539030307423672638833522796630859375;1.0645797575868669593290860575507394969463348388671875;0.11810308490167364947609485170687548816204071044921875;-0.372071517987673849869878495155717246234416961669921875;-0.283477389236025445473643458171864040195941925048828125;0.9522324461670808037894175868132151663303375244140625;-1.1304134726978232183824957246542908251285552978515625;0.068293414585643141823112500787829048931598663330078125]
      mask Display: e = 0.06;c1 = [120 150 230]/255;c2 = ([120 150 230]+0)/383;c3 = ([120 150 230]+128)/383;patch([0 1 1 0],[0 0 1 1],c1);patch([0 1 1 1-e 1-e 0+e],[0 0 1 1-e 0+e 0+e],c2);patch([0 0 1 1-e 0+e 0+e],[0 1 1 1-e 1-e 0+e],c3);plot([0 1 1 0 0],[0 0 1 1 0]);disp('Weights');
  "IW{1,1}(5,:)'" : Constant  Value=[0.9402560928758985081543642081669531762599945068359375;-0.4066332967723680358318461003364063799381256103515625;0.26533136534984647081358843934140168130397796630859375;-0.477720029105056898099945783542352728545665740966796875;0.590134246153905195342304068617522716522216796875;-0.2572731608379810186448821696103550493717193603515625;0.316808760305900827258795970919891260564327239990234375;-1.1948930430904469712771742706536315381526947021484375;-1.213821179879751799290943381492979824542999267578125]
      mask Display: e = 0.06;c1 = [120 150 230]/255;c2 = ([120 150 230]+0)/383;c3 = ([120 150 230]+128)/383;patch([0 1 1 0],[0 0 1 1],c1);patch([0 1 1 1-e 1-e 0+e],[0 0 1 1-e 0+e 0+e],c2);patch([0 0 1 1-e 0+e 0+e],[0 1 1 1-e 1-e 0+e],c3);plot([0 1 1 0 0],[0 0 1 1 0]);disp('Weights');
  "IW{1,1}(50,:)'" : Constant  Value=[0.293937452932246323644704943944816477596759796142578125;-0.295183647305805429983394105875049717724323272705078125;1.2902606046384252902470279877888970077037811279296875;-0.2355898506475904152779321520938538014888763427734375;-1.0034426640904696714784449795843102037906646728515625;-0.78492621273633300660321765462867915630340576171875;-0.75251005841944518248709528052131645381450653076171875;-0.05214153429156154206935980255366303026676177978515625;-0.7796342604648012208912177811725996434688568115234375]
      mask Display: e = 0.06;c1 = [120 150 230]/255;c2 = ([120 150 230]+0)/383;c3 = ([120 150 230]+128)/383;patch([0 1 1 0],[0 0 1 1],c1);patch([0 1 1 1-e 1-e 0+e],[0 0 1 1-e 0+e 0+e],c2);patch([0 0 1 1-e 0+e 0+e],[0 1 1 1-e 1-e 0+e],c3);plot([0 1 1 0 0],[0 0 1 1 0]);disp('Weights');
  "IW{1,1}(6,:)'" : Constant  Value=[-0.286526770121102003496815768812666647136211395263671875;0.7444765059505495941039043827913701534271240234375;-0.5900379005736453574826327894697897136211395263671875;-0.85689718588324137460432439183932729065418243408203125;0.72605198823461025714465222336002625524997711181640625;0.51071850901931881150375147626618854701519012451171875;0.46045994753051633363583050595480017364025115966796875;-1.3878827643061411034608454428962431848049163818359375;-1.3924669454928799705584196999552659690380096435546875]
      mask Display: e = 0.06;c1 = [120 150 230]/255;c2 = ([120 150 230]+0)/383;c3 = ([120 150 230]+128)/383;patch([0 1 1 0],[0 0 1 1],c1);patch([0 1 1 1-e 1-e 0+e],[0 0 1 1-e 0+e 0+e],c2);patch([0 0 1 1-e 0+e 0+e],[0 1 1 1-e 1-e 0+e],c3);plot([0 1 1 0 0],[0 0 1 1 0]);disp('Weights');
  "IW{1,1}(7,:)'" : Constant  Value=[0.8273960718063886332629408570937812328338623046875;-1.0953288896866146817643539179698564112186431884765625;-0.80276876675725772347647080096066929399967193603515625;0.399921082458345178434200306583079509437084197998046875;-1.1376169512115186233103258928167633712291717529296875;-0.1662365018389222459660459207952953875064849853515625;0.11489584072191126595807730836895643733441829681396484375;0.08027062508521613792833448997043888084590435028076171875;-0.464523135947423393421473747366690076887607574462890625]
      mask Display: e = 0.06;c1 = [120 150 230]/255;c2 = ([120 150 230]+0)/383;c3 = ([120 150 230]+128)/383;patch([0 1 1 0],[0 0 1 1],c1);patch([0 1 1 1-e 1-e 0+e],[0 0 1 1-e 0+e 0+e],c2);patch([0 0 1 1-e 0+e 0+e],[0 1 1 1-e 1-e 0+e],c3);plot([0 1 1 0 0],[0 0 1 1 0]);disp('Weights');
  "IW{1,1}(8,:)'" : Constant  Value=[-0.1903599507540090496338081038629752583801746368408203125;0.315697508931002290832878998116939328610897064208984375;0.7403249684598762758724888044525869190692901611328125;1.1307095649380893842561590645345859229564666748046875;1.0358386395770582399933346096077002584934234619140625;-0.20497312931890931952949586047907359898090362548828125;-0.390062432887791910030017561439308337867259979248046875;0.8860302300443814171870826612575910985469818115234375;0.92268983444323804388176313295844011008739471435546875]
      mask Display: e = 0.06;c1 = [120 150 230]/255;c2 = ([120 150 230]+0)/383;c3 = ([120 150 230]+128)/383;patch([0 1 1 0],[0 0 1 1],c1);patch([0 1 1 1-e 1-e 0+e],[0 0 1 1-e 0+e 0+e],c2);patch([0 0 1 1-e 0+e 0+e],[0 1 1 1-e 1-e 0+e],c3);plot([0 1 1 0 0],[0 0 1 1 0]);disp('Weights');
  "IW{1,1}(9,:)'" : Constant  Value=[0.7760224271093842940416607234510593116283416748046875;0.288576184201353613811846798853366635739803314208984375;-0.295052908172059591418445734234410338103771209716796875;-0.250090362485558437288801769682322628796100616455078125;-0.446071785205032711463246641869773156940937042236328125;-0.9601525700366233539995164392166770994663238525390625;0.674240184022305566458044268074445426464080810546875;-0.8192177013571058097340937820263206958770751953125;1.0603357049241228793334812507964670658111572265625]
      mask Display: e = 0.06;c1 = [120 150 230]/255;c2 = ([120 150 230]+0)/383;c3 = ([120 150 230]+128)/383;patch([0 1 1 0],[0 0 1 1],c1);patch([0 1 1 1-e 1-e 0+e],[0 0 1 1-e 0+e 0+e],c2);patch([0 0 1 1-e 0+e 0+e],[0 1 1 1-e 1-e 0+e],c3);plot([0 1 1 0 0],[0 0 1 1 0]);disp('Weights');
  Mux : Mux  Inputs=50
      mask Display: e = 0.06;c1 = [120 150 230]/255;c2 = ([120 150 230]+0)/383;c3 = ([120 150 230]+128)/383;patch([0 1 1 0],[0 0 1 1],c1);patch([0 1 1 1-e 1-e 0+e],[0 0 1 1-e 0+e 0+e],c2);patch([0 0 1 1-e 0+e 0+e],[0 1 1 1-e 1-e 0+e],c3);plot([0 1 1 0 0],[0 0 1 1 0]);disp('Mux');
  dotprod{1..50} (50 alike) : neural/Weight Functions/dotprod
  "iz{1,1}" : Outport
      mask Display: e = 0.06;c1 = [120 230 180]/255;c2 = ([120 230 180]+0)/(256+128);c3 = ([120 230 180]+128)/(256+128);patch([0 1 1 0],[0 0 1 1],c1);patch([0 1 1 1-e 1-e 0+e],[0 0 1 1-e 0+e 0+e],c2);patch([0 0 1 1-e 0+e 0+e],[0 1 1 1-e 1-e 0+e],c3);plot([0 1 1 0 0],[0 0 1 1 0]);
  wires:
  "IW{1,1}(1,:)'"/1 -> dotprod1/1
  "pd{1,1}"/1 -> dotprod1/2, dotprod2/2, dotprod3/2, dotprod4/2, dotprod5/2, dotprod6/2, dotprod7/2, dotprod8/2, dotprod9/2, dotprod10/2, dotprod11/2, dotprod12/2, dotprod13/2, dotprod14/2, dotprod15/2, dotprod16/2, dotprod17/2, dotprod18/2, dotprod19/2, dotprod20/2, dotprod21/2, dotprod22/2, dotprod23/2, dotprod24/2, dotprod25/2, dotprod26/2, dotprod27/2, dotprod28/2, dotprod29/2, dotprod30/2, dotprod31/2, dotprod32/2, dotprod33/2, dotprod34/2, dotprod35/2, dotprod36/2, dotprod37/2, dotprod38/2, dotprod39/2, dotprod40/2, dotprod41/2, dotprod42/2, dotprod43/2, dotprod44/2, dotprod45/2, dotprod46/2, dotprod47/2, dotprod48/2, dotprod49/2, dotprod50/2
  dotprod1/1 -> Mux/1
  "IW{1,1}(2,:)'"/1 -> dotprod2/1
  dotprod2/1 -> Mux/2
  "IW{1,1}(3,:)'"/1 -> dotprod3/1
  dotprod3/1 -> Mux/3
  "IW{1,1}(4,:)'"/1 -> dotprod4/1
  dotprod4/1 -> Mux/4
  "IW{1,1}(5,:)'"/1 -> dotprod5/1
  dotprod5/1 -> Mux/5
  "IW{1,1}(6,:)'"/1 -> dotprod6/1
  dotprod6/1 -> Mux/6
  "IW{1,1}(7,:)'"/1 -> dotprod7/1
  dotprod7/1 -> Mux/7
  "IW{1,1}(8,:)'"/1 -> dotprod8/1
  dotprod8/1 -> Mux/8
  "IW{1,1}(9,:)'"/1 -> dotprod9/1
  dotprod9/1 -> Mux/9
  "IW{1,1}(10,:)'"/1 -> dotprod10/1
  dotprod10/1 -> Mux/10
  "IW{1,1}(11,:)'"/1 -> dotprod11/1
  dotprod11/1 -> Mux/11
  "IW{1,1}(12,:)'"/1 -> dotprod12/1
  dotprod12/1 -> Mux/12
  "IW{1,1}(13,:)'"/1 -> dotprod13/1
  dotprod13/1 -> Mux/13
  "IW{1,1}(14,:)'"/1 -> dotprod14/1
  dotprod14/1 -> Mux/14
  "IW{1,1}(15,:)'"/1 -> dotprod15/1
  dotprod15/1 -> Mux/15
  "IW{1,1}(16,:)'"/1 -> dotprod16/1
  dotprod16/1 -> Mux/16
  "IW{1,1}(17,:)'"/1 -> dotprod17/1
  dotprod17/1 -> Mux/17
  "IW{1,1}(18,:)'"/1 -> dotprod18/1
  dotprod18/1 -> Mux/18
  "IW{1,1}(19,:)'"/1 -> dotprod19/1
  dotprod19/1 -> Mux/19
  "IW{1,1}(20,:)'"/1 -> dotprod20/1
  dotprod20/1 -> Mux/20
  "IW{1,1}(21,:)'"/1 -> dotprod21/1
  dotprod21/1 -> Mux/21
  "IW{1,1}(22,:)'"/1 -> dotprod22/1
  dotprod22/1 -> Mux/22
  "IW{1,1}(23,:)'"/1 -> dotprod23/1
  dotprod23/1 -> Mux/23
  "IW{1,1}(24,:)'"/1 -> dotprod24/1
  dotprod24/1 -> Mux/24
  "IW{1,1}(25,:)'"/1 -> dotprod25/1
  dotprod25/1 -> Mux/25
  "IW{1,1}(26,:)'"/1 -> dotprod26/1
  dotprod26/1 -> Mux/26
  "IW{1,1}(27,:)'"/1 -> dotprod27/1
  dotprod27/1 -> Mux/27
  "IW{1,1}(28,:)'"/1 -> dotprod28/1
  dotprod28/1 -> Mux/28
  "IW{1,1}(29,:)'"/1 -> dotprod29/1
  dotprod29/1 -> Mux/29
  "IW{1,1}(30,:)'"/1 -> dotprod30/1
  dotprod30/1 -> Mux/30
  "IW{1,1}(31,:)'"/1 -> dotprod31/1
  dotprod31/1 -> Mux/31
  "IW{1,1}(32,:)'"/1 -> dotprod32/1
  dotprod32/1 -> Mux/32
  "IW{1,1}(33,:)'"/1 -> dotprod33/1
  dotprod33/1 -> Mux/33
  "IW{1,1}(34,:)'"/1 -> dotprod34/1
  dotprod34/1 -> Mux/34
  "IW{1,1}(35,:)'"/1 -> dotprod35/1
  dotprod35/1 -> Mux/35
  "IW{1,1}(36,:)'"/1 -> dotprod36/1
  dotprod36/1 -> Mux/36
  "IW{1,1}(37,:)'"/1 -> dotprod37/1
  dotprod37/1 -> Mux/37
  "IW{1,1}(38,:)'"/1 -> dotprod38/1
  dotprod38/1 -> Mux/38
  "IW{1,1}(39,:)'"/1 -> dotprod39/1
  dotprod39/1 -> Mux/39
  "IW{1,1}(40,:)'"/1 -> dotprod40/1
  dotprod40/1 -> Mux/40
  "IW{1,1}(41,:)'"/1 -> dotprod41/1
  dotprod41/1 -> Mux/41
  "IW{1,1}(42,:)'"/1 -> dotprod42/1
  dotprod42/1 -> Mux/42
  "IW{1,1}(43,:)'"/1 -> dotprod43/1
  dotprod43/1 -> Mux/43
  "IW{1,1}(44,:)'"/1 -> dotprod44/1
  dotprod44/1 -> Mux/44
  "IW{1,1}(45,:)'"/1 -> dotprod45/1
  dotprod45/1 -> Mux/45
  "IW{1,1}(46,:)'"/1 -> dotprod46/1
  dotprod46/1 -> Mux/46
  "IW{1,1}(47,:)'"/1 -> dotprod47/1
  dotprod47/1 -> Mux/47
  "IW{1,1}(48,:)'"/1 -> dotprod48/1
  dotprod48/1 -> Mux/48
  "IW{1,1}(49,:)'"/1 -> dotprod49/1
  dotprod49/1 -> Mux/49
  "IW{1,1}(50,:)'"/1 -> dotprod50/1
  dotprod50/1 -> Mux/50
  Mux/1 -> "iz{1,1}"/1

== system control_system/Function Fitting Neural Network3/Layer 2/Delays 1 ==
  "p{2}" : Inport  PortDimensions=50  SampleTime=0.1
      mask Display: e = 0.06;c1 = [120 230 180]/255;c2 = ([120 230 180]+0)/(256+128);c3 = ([120 230 180]+128)/(256+128);patch([0 1 1 0],[0 0 1 1],c1);patch([0 1 1 1-e 1-e 0+e],[0 0 1 1-e 0+e 0+e],c2);patch([0 0 1 1-e 0+e 0+e],[0 1 1 1-e 1-e 0+e],c3);plot([0 1 1 0 0],[0 0 1 1 0]);
  mux : Mux  Inputs=1
      mask Display: e = 0.06;c1 = [120 150 230]/255;c2 = ([120 150 230]+0)/383;c3 = ([120 150 230]+128)/383;patch([0 1 1 0],[0 0 1 1],c1);patch([0 1 1 1-e 1-e 0+e],[0 0 1 1-e 0+e 0+e],c2);patch([0 0 1 1-e 0+e 0+e],[0 1 1 1-e 1-e 0+e],c3);plot([0 1 1 0 0],[0 0 1 1 0]);disp('Mux')
  "pd{2,1}" : Outport
      mask Display: e = 0.06;c1 = [120 230 180]/255;c2 = ([120 230 180]+0)/(256+128);c3 = ([120 230 180]+128)/(256+128);patch([0 1 1 0],[0 0 1 1],c1);patch([0 1 1 1-e 1-e 0+e],[0 0 1 1-e 0+e 0+e],c2);patch([0 0 1 1-e 0+e 0+e],[0 1 1 1-e 1-e 0+e],c3);plot([0 1 1 0 0],[0 0 1 1 0]);
  wires:
  "p{2}"/1 -> mux/1
  mux/1 -> "pd{2,1}"/1
